simulink model "telemetrySources"  (Simulink 6.6)
settings: Solver=ode3  StartTime=0.0  StopTime=time(end)  FixedStep=0.01  RelTol=1e-3
values from neighbouring files (symbols this model uses):
  baseHeight = GPS_hil(1,3)    [telemetryToHil.m]
  GS_location = [0 36.9898376464844 -122.051963806152]    [telemetryToHil.m]
  ISA_rho0 = 1.225    [Taxi_Var.m]
  T = 0.01    [Taxi_Var.m]
undefined symbols (not defined in the file or in its folder): baroMeanTemp, baroOffset, baroScale, baroTempK, baseTemp, gaind, lapseRate, magMeanTemp, magOffset, magScale, magTempK, pitMeanTemp, pitotOffset, pitotScale, pitTempK, polesd, tempOffset, tempScale, zerosd
libraries: simulink x4, aerolibconvert2 x1
settings Model: Creator=Administrator  LastModifiedBy=Administrator

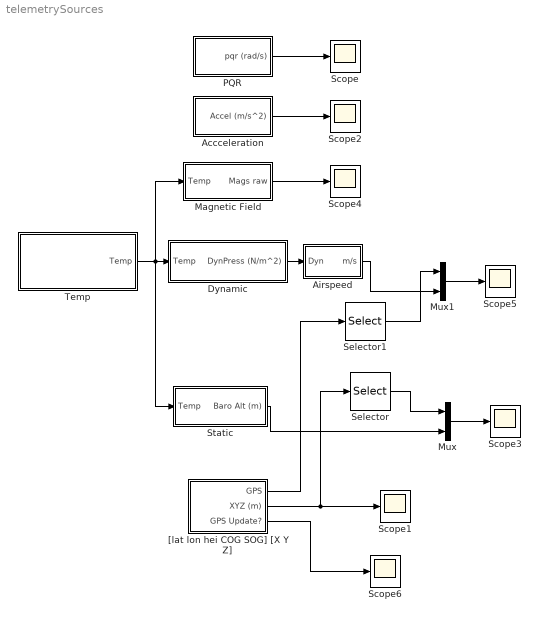
== system telemetrySources ==
  Accceleration : Subsystem
  Airspeed : Subsystem
  Dynamic : Subsystem
  Magnetic Field : Subsystem
  Mux : Mux  Inputs=2
  Mux1 : Mux  Inputs=2
  PQR : Subsystem
  Scope{,1..6} (7 alike) : Scope
      Scope1 settings: TimeRange=60  YMin=-1500  YMax=1500
      Scope2 settings: SaveName=ScopeData2
      Scope3 settings: TimeRange=1540.45  YMin=70  YMax=260  SaveName=ScopeData3
      Scope4 settings: SaveName=ScopeData4
      Scope5 settings: TimeRange=500  YMin=-40  YMax=30  SaveName=ScopeData5
      Scope6 settings: TimeRange=60  YMin=-1500  YMax=1500  SaveName=ScopeData6
  Selector : Selector  IndexOptions=Index vector (dialog)  Indices=[3]  OutputSizes=1  InputPortWidth=3
  Selector1 : Selector  IndexOptions=Index vector (dialog)  Indices=[5]  OutputSizes=1  InputPortWidth=5
  Static : Subsystem
  Temp : Subsystem
  "[lat lon hei COG SOG] [X Y Z]" : Subsystem
  wires:
  PQR/1(pqr (rad/s)) -> Scope/1
  "[lat lon hei COG SOG] [X Y Z]"/2(XYZ (m)) -> Selector/1, Scope1/1
  Accceleration/1(Accel (m/s^2)) -> Scope2/1
  Static/1(Baro Alt (m)) -> Mux/2
  Mux/1 -> Scope3/1
  Selector/1 -> Mux/1
  Magnetic Field/1(Mags raw) -> Scope4/1
  Temp/1(Temp) -> Magnetic Field/1(Temp), Dynamic/1(Temp), Static/1(Temp)
  Dynamic/1(DynPress (N/m^2)) -> Airspeed/1(Dyn)
  "[lat lon hei COG SOG] [X Y Z]"/1(GPS) -> Selector1/1
  Selector1/1 -> Mux1/1
  Mux1/1 -> Scope5/1
  Airspeed/1(m/s) -> Mux1/2
  "[lat lon hei COG SOG] [X Y Z]"/3(GPS Update?) -> Scope6/1

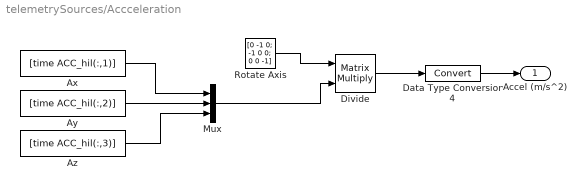
== system telemetrySources/Accceleration ==
  Ax : FromWorkspace  VariableName=[time ACC_hil(:,1)]  SampleTime=0.01  OutputAfterFinalValue=Setting to zero
  Ay : FromWorkspace  VariableName=[time ACC_hil(:,2)]  SampleTime=0.01  OutputAfterFinalValue=Setting to zero
  Az : FromWorkspace  VariableName=[time ACC_hil(:,3)]  SampleTime=0.01  OutputAfterFinalValue=Setting to zero
  Data Type Conversion4 : DataTypeConversion  OutDataTypeMode=single
  Divide : Product  Multiplication=Matrix(*)  OutScaling=2^-10
  Mux : Mux  Inputs=3
  Rotate Axis : Constant  Value=[0 -1 0; -1 0 0; 0 0 -1]
  Accel (m/s^2) : Outport
  wires:
  Az/1 -> Mux/3
  Ay/1 -> Mux/2
  Ax/1 -> Mux/1
  Data Type Conversion4/1 -> Accel (m/s^2)/1
  Rotate Axis/1 -> Divide/1
  Mux/1 -> Divide/2
  Divide/1 -> Data Type Conversion4/1

== system telemetrySources/Airspeed ==
  Dyn : Inport
  Gain : Gain  Gain=2/ISA_rho0
  Math Function : Math  Operator=sqrt  SaturateOnIntegerOverflow=on
  "[0.001  2000]" : Saturate  UpperLimit=2000  LowerLimit=0.001
  m/s : Outport
  wires:
  Gain/1 -> "[0.001  2000]"/1
  Dyn/1 -> Gain/1
  Math Function/1 -> m/s/1
  "[0.001  2000]"/1 -> Math Function/1

== system telemetrySources/Dynamic ==
  Temp : Inport
  Data Type Conversion1 : DataTypeConversion  OutDataTypeMode=single
  Dyn : FromWorkspace  VariableName=[time DYN_hil(:,1)]  SampleTime=0.01  OutputAfterFinalValue=Setting to zero
  Low Pass1 : Subsystem  mask(DiscretizedZeroPole){Zeros=[], Poles=[-30], Gain=30, AbsTol=auto, SampleTime=T, method=tustin, Wc=1}
      mask prompts: Zeros "Zeros (enter in s-main:)"; Poles "Poles (enter in s-domain:)"; Gain "Gain (enter in s-domain:)"; AbsTol "Absolute tolerance:"; SampleTime "Sample time:"; Wc "Critical Frequency (Hz):"
      mask help: Continuous mask uses c2d to transform parameters onto the Discrete Zero-Pole block inside.
      mask init:
      | st=SampleTime;
      | if length(st)>1
      |     st=SampleTime(1);
      | end
      | if(st>0)
      |     [zerosd,polesd,gaind] = sldiscutil('disczpk', {st,method,Wc,Zeros,Poles,Gain});
      | end	
      | s = get_param(gcb,'maskvalues');
      | zeross = s{1};
      | poless = s{2};
      | gainss = s{3};
      | %zerosc = eval(zeross);
      | %polesc = eval(poless);
      | %gainsc = eval(gainss);
      | sldiscutil('initzpkmask', st);
      | if(st==0)
      | set_param([gcb '/Zero Pole'], 'AbsoluteTolerance', AbsTol);
      | end
      mask StyleString: edit,edit,edit,edit,edit,popup(zoh|foh|tustin|prewarp|matched),edit
      mask CallbackString: |||||hidecrit|
      mask Display:
      | droots(zeross,poless,gainss)
      | text( 0.5, 1.0, method, 'verticalAlignment','top')
  Pitot Unit Conversion : Subsystem  mask{bias=pitotOffset, gains=pitotScale}
      mask prompts: bias "Initial Bias"; gains "Initial Gains"
      mask help: Convert Analog readings to units
  Pitot Temp Compensation : Subsystem  mask{alpha=pitTempK, tempMean=pitMeanTemp}
      mask prompts: alpha "Tempearature Coeficient (K_t)"; tempMean "Calibration Temperature Mean (T_avg)"
      mask help:
      | This block implements a temperature compensation. It implmements the following equation:
      |
      | M_tc = M_raw - K_t(T - T_avg)
  DynPress (N/m^2) : Outport
  wires:
  Dyn/1 -> Low Pass1/1(In1)
  Low Pass1/1(Out1) -> Data Type Conversion1/1
  Data Type Conversion1/1 -> Pitot Unit Conversion/1(Raw)
  Pitot Temp Compensation/1(Comp) -> DynPress (N/m^2)/1
  Temp/1 -> Pitot Temp Compensation/2(Temp Raw)
  Pitot Unit Conversion/1(Comp) -> Pitot Temp Compensation/1(Raw)

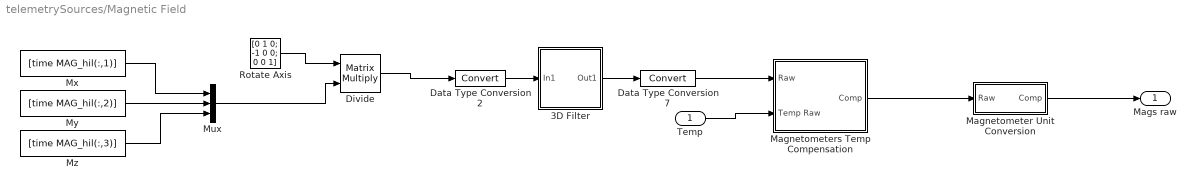
== system telemetrySources/Magnetic Field ==
  Temp : Inport
  3D Filter : Subsystem  AncestorBlock=SLUGS_Library/Singnal Routing & Conditioning/3D Filter  RTWFcnName=TustinFilter3D  mask{zval=[], pval=-150, kval=150, TSample=0.01}
      mask prompts: zval "Zeros"; pval "Poles"; kval "Gains"; TSample "Sample Time"
      settings: RTWFcnNameOpts=User specified  RTWFileNameOpts=Use function name
      mask Display:
      | droots(zval,pval,kval)
      | port_label('input',1,'3D')
  Data Type Conversion2 : DataTypeConversion  OutDataTypeMode=double
  Data Type Conversion7 : DataTypeConversion  OutDataTypeMode=single
  Divide : Product  Multiplication=Matrix(*)  OutScaling=2^-10
  Magnetometer Unit Conversion : Subsystem  mask{bias=magOffset, gains=magScale}
      mask prompts: bias "Initial Bias"; gains "Initial Gains"
      mask help: Convert Analog readings to units
  Magnetometers Temp Compensation : Subsystem  mask{alpha=magTempK, tempMean=magMeanTemp}
      mask prompts: alpha "Tempearature Coeficient (K_t)"; tempMean "Calibration Temperature Mean (T_avg)"
      mask help:
      | This block implements a temperature compensation. It implmements the following equation:
      |
      | M_tc = M_raw - K_t(T - T_avg)
  Mux : Mux  Inputs=3
  Mx : FromWorkspace  VariableName=[time MAG_hil(:,1)]  SampleTime=0.01  OutputAfterFinalValue=Setting to zero
  My : FromWorkspace  VariableName=[time MAG_hil(:,2)]  SampleTime=0.01  OutputAfterFinalValue=Setting to zero
  Mz : FromWorkspace  VariableName=[time MAG_hil(:,3)]  SampleTime=0.01  OutputAfterFinalValue=Setting to zero
  Rotate Axis : Constant  Value=[0 1 0; -1 0 0; 0 0 1]
  Mags raw : Outport
  wires:
  Mx/1 -> Mux/1
  My/1 -> Mux/2
  Mz/1 -> Mux/3
  Rotate Axis/1 -> Divide/1
  Mux/1 -> Divide/2
  Data Type Conversion2/1 -> 3D Filter/1(In1)
  3D Filter/1(Out1) -> Data Type Conversion7/1
  Data Type Conversion7/1 -> Magnetometers Temp Compensation/1(Raw)
  Magnetometers Temp Compensation/1(Comp) -> Magnetometer Unit Conversion/1(Raw)
  Divide/1 -> Data Type Conversion2/1
  Temp/1 -> Magnetometers Temp Compensation/2(Temp Raw)
  Magnetometer Unit Conversion/1(Comp) -> Mags raw/1

== system telemetrySources/PQR ==
  Data Type Conversion1 : DataTypeConversion  OutDataTypeMode=single
  Divide : Product  Multiplication=Matrix(*)  OutScaling=2^-10
  Mux : Mux  Inputs=3
  Rotate Axis : Constant  Value=[0 -1 0; -1 0 0; 0 0 -1]
  p : FromWorkspace  VariableName=[time PQR_hil(:,1)]  SampleTime=0.01  OutputAfterFinalValue=Setting to zero
  q : FromWorkspace  VariableName=[time PQR_hil(:,2)]  SampleTime=0.01  OutputAfterFinalValue=Setting to zero
  r : FromWorkspace  VariableName=[time PQR_hil(:,3)]  SampleTime=0.01  OutputAfterFinalValue=Setting to zero
  pqr (rad/s) : Outport
  wires:
  p/1 -> Mux/1
  q/1 -> Mux/2
  r/1 -> Mux/3
  Data Type Conversion1/1 -> pqr (rad/s)/1
  Rotate Axis/1 -> Divide/1
  Mux/1 -> Divide/2
  Divide/1 -> Data Type Conversion1/1

== system telemetrySources/Static ==
  Temp : Inport
  Baro Altimeter : Subsystem
  Baro Temp Compensation : Subsystem  mask{alpha=baroTempK, tempMean=baroMeanTemp}
      mask prompts: alpha "Tempearature Coeficient (K_t)"; tempMean "Calibration Temperature Mean (T_avg)"
      mask help:
      | This block implements a temperature compensation. It implmements the following equation:
      |
      | M_tc = M_raw - K_t(T - T_avg)
  Barometer Unit Conversion : Subsystem  mask{bias=baroOffset, gains=baroScale}
      mask prompts: bias "Initial Bias"; gains "Initial Gains"
      mask help: Convert Analog readings to units
  Data Type Conversion1 : DataTypeConversion  OutDataTypeMode=single
  Dyn : FromWorkspace  VariableName=[time STA_hil(:,1)]  SampleTime=0.01  OutputAfterFinalValue=Setting to zero
  Low Pass1 : Subsystem  mask(DiscretizedZeroPole){Zeros=[], Poles=[-1], Gain=1, AbsTol=auto, SampleTime=T, method=tustin, Wc=1}
      mask prompts: Zeros "Zeros (enter in s-main:)"; Poles "Poles (enter in s-domain:)"; Gain "Gain (enter in s-domain:)"; AbsTol "Absolute tolerance:"; SampleTime "Sample time:"; Wc "Critical Frequency (Hz):"
      mask help: Continuous mask uses c2d to transform parameters onto the Discrete Zero-Pole block inside.
      mask init: same as telemetrySources/Dynamic/Low Pass1
      mask StyleString: edit,edit,edit,edit,edit,popup(zoh|foh|tustin|prewarp|matched),edit
      mask CallbackString: |||||hidecrit|
      mask Display:
      | droots(zeross,poless,gainss)
      | text( 0.5, 1.0, method, 'verticalAlignment','top')
  Baro Alt (m) : Outport
  wires:
  Low Pass1/1(Out1) -> Data Type Conversion1/1
  Dyn/1 -> Low Pass1/1(In1)
  Baro Altimeter/1(Altitude) -> Baro Alt (m)/1
  Barometer Unit Conversion/1(Comp) -> Baro Temp Compensation/1(Raw)
  Baro Temp Compensation/1(Comp) -> Baro Altimeter/1(Static Raw)
  Data Type Conversion1/1 -> Barometer Unit Conversion/1(Raw)
  Temp/1 -> Baro Temp Compensation/2(Temp Raw)

== system telemetrySources/Temp ==
  Data Type Conversion5 : DataTypeConversion  OutDataTypeMode=single
  Dyn : FromWorkspace  VariableName=[time TEM_hil(:,1)]  SampleTime=0.01  OutputAfterFinalValue=Setting to zero
  Low Pass8 : Subsystem  mask(DiscretizedZeroPole){Zeros=[], Poles=[-5], Gain=5, AbsTol=auto, SampleTime=T, method=tustin, Wc=1}
      mask prompts: Zeros "Zeros (enter in s-main:)"; Poles "Poles (enter in s-domain:)"; Gain "Gain (enter in s-domain:)"; AbsTol "Absolute tolerance:"; SampleTime "Sample time:"; Wc "Critical Frequency (Hz):"
      mask help: Continuous mask uses c2d to transform parameters onto the Discrete Zero-Pole block inside.
      mask init: same as telemetrySources/Dynamic/Low Pass1
      mask StyleString: edit,edit,edit,edit,edit,popup(zoh|foh|tustin|prewarp|matched),edit
      mask CallbackString: |||||hidecrit|
      mask Display:
      | droots(zeross,poless,gainss)
      | text( 0.5, 1.0, method, 'verticalAlignment','top')
  Thermistor Unit Conversion : Subsystem  mask{bias=tempOffset, gains=tempScale}
      mask prompts: bias "Initial Bias"; gains "Initial Gains"
      mask help: Convert Analog readings to units
  Temp : Outport
  wires:
  Dyn/1 -> Low Pass8/1(In1)
  Low Pass8/1(Out1) -> Data Type Conversion5/1
  Thermistor Unit Conversion/1(Comp) -> Temp/1
  Data Type Conversion5/1 -> Thermistor Unit Conversion/1(Raw)

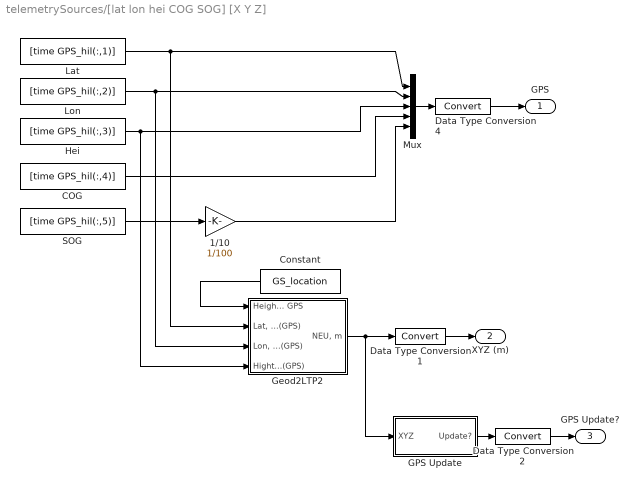
== system telemetrySources/[lat lon hei COG SOG] [X Y Z] ==
  1/10 : Gain  Gain=1/100
  COG : FromWorkspace  VariableName=[time GPS_hil(:,4)]  SampleTime=0.01  OutputAfterFinalValue=Setting to zero
  Constant : Constant  Orientation=left  Value=GS_location
  Data Type Conversion1 : DataTypeConversion  OutDataTypeMode=single
  Data Type Conversion2 : DataTypeConversion  OutDataTypeMode=uint8
  Data Type Conversion4 : DataTypeConversion  OutDataTypeMode=single
  GPS Update : Subsystem  mask{T=0.01}
      mask prompts: T "Sample Time"
  Geod2LTP2 : Subsystem
      mask Description:
      | This block provides transformation of the Geodetic coordinates
      | to the LTP coorinate system. The block uses two consecutive transformations
      | (Geodetic -> ECEF ->LTP).
      | Geodetic coordinates of the LTP origin should also be predetermined.
      mask Help: Oops!
      mask Display: plot(0,0,100,100,[45,40,35,40,40],[85,95,85,95,40],[85,95,85,95,40],[35,40,45,40,40],[60,40,10,20,10,14],[70,40,10,13,10,20],[56,45],[70,70],[60,60],[50,60],[60,60],[30,40],[50,60],[20,20],[30,40],[20,20],[45,55],[35,25],[75,65],[35,25])
  Hei : FromWorkspace  VariableName=[time GPS_hil(:,3)]  SampleTime=0.01  OutputAfterFinalValue=Setting to zero
  Lat : FromWorkspace  VariableName=[time GPS_hil(:,1)]  SampleTime=0.01  OutputAfterFinalValue=Setting to zero
  Lon : FromWorkspace  VariableName=[time GPS_hil(:,2)]  SampleTime=0.01  OutputAfterFinalValue=Setting to zero
  Mux : Mux  Inputs=5
  SOG : FromWorkspace  VariableName=[time GPS_hil(:,5)]  SampleTime=0.01  OutputAfterFinalValue=Setting to zero
  GPS : Outport
  XYZ (m) : Outport  Port=2
  GPS Update? : Outport  Port=3
  wires:
  Lat/1 -> Mux/1, Geod2LTP2/2("Lat, deg(GPS)")
  Lon/1 -> Mux/2, Geod2LTP2/3("Lon, deg(GPS)")
  Hei/1 -> Mux/3, Geod2LTP2/4(Hight,m(GPS))
  Mux/1 -> Data Type Conversion4/1
  COG/1 -> Mux/4
  SOG/1 -> 1/10/1
  Constant/1 -> Geod2LTP2/1("Height, Lat, Lon Initials from GPS")
  Geod2LTP2/1("NEU, m") -> GPS Update/1(XYZ), Data Type Conversion1/1
  GPS Update/1(Update?) -> Data Type Conversion2/1
  1/10/1 -> Mux/5
  Data Type Conversion4/1 -> GPS/1
  Data Type Conversion1/1 -> XYZ (m)/1
  Data Type Conversion2/1 -> GPS Update?/1

== system telemetrySources/Dynamic/Low Pass1 ==
  In1 : Inport
  Discrete Zero-Pole : DiscreteZeroPole  Zeros=zerosd  Poles=polesd  Gain=gaind  SampleTime=SampleTime
  Out1 : Outport
  wires:
  In1/1 -> Discrete Zero-Pole/1
  Discrete Zero-Pole/1 -> Out1/1

== system telemetrySources/Dynamic/Pitot Unit Conversion ==
  Raw : Inport
  Bias : Constant  Value=bias  OutDataTypeMode=single
  Divide : Product  OutDataTypeMode=single  OutScaling=2^-10
  Gains : Constant  Value=gains  OutDataTypeMode=single
  Sum : Sum  Inputs=|++  OutDataTypeMode=single
  Comp : Outport
  wires:
  Bias/1 -> Sum/2
  Raw/1 -> Divide/2
  Gains/1 -> Divide/1
  Divide/1 -> Sum/1
  Sum/1 -> Comp/1

== system telemetrySources/Dynamic/Pitot Temp Compensation ==
  Raw : Inport
  Temp Raw : Inport  Port=2
  Divide1 : Product  OutDataTypeMode=single  OutScaling=2^-10
  Mean Temperature for Calibration : Constant  Value=tempMean  OutDataTypeMode=single
  Sum1 : Sum  Inputs=|+-  OutDataTypeMode=single
  Sum2 : Sum  Inputs=|+-  OutDataTypeMode=single
  gains : Constant  Value=alpha  OutDataTypeMode=single
  Comp : Outport
  wires:
  Mean Temperature for Calibration/1 -> Sum1/2
  Raw/1 -> Sum2/1
  Temp Raw/1 -> Sum1/1
  Sum1/1 -> Divide1/2
  gains/1 -> Divide1/1
  Divide1/1 -> Sum2/2
  Sum2/1 -> Comp/1

== system telemetrySources/Magnetic Field/3D Filter ==
  In1 : Inport
  Demux : Demux  Outputs=3
  Filter1 : Subsystem  mask(DiscretizedZeroPole){Zeros=zval, Poles=pval, Gain=kval, AbsTol=auto, SampleTime=TSample, method=tustin, Wc=1}
      mask prompts: Zeros "Zeros (enter in s-main:)"; Poles "Poles (enter in s-domain:)"; Gain "Gain (enter in s-domain:)"; AbsTol "Absolute tolerance:"; SampleTime "Sample time:"; Wc "Critical Frequency (Hz):"
      mask help: Continuous mask uses c2d to transform parameters onto the Discrete Zero-Pole block inside.
      mask init: same as telemetrySources/Dynamic/Low Pass1
      mask StyleString: edit,edit,edit,edit,edit,popup(zoh|foh|tustin|prewarp|matched),edit
      mask CallbackString: |||||hidecrit|
      mask Display:
      | droots(zeross,poless,gainss)
      | text( 0.5, 1.0, method, 'verticalAlignment','top')
  Filter2 : Subsystem  mask(DiscretizedZeroPole){Zeros=zval, Poles=pval, Gain=kval, AbsTol=auto, SampleTime=TSample, method=tustin, Wc=1}
      mask prompts: Zeros "Zeros (enter in s-main:)"; Poles "Poles (enter in s-domain:)"; Gain "Gain (enter in s-domain:)"; AbsTol "Absolute tolerance:"; SampleTime "Sample time:"; Wc "Critical Frequency (Hz):"
      mask help: Continuous mask uses c2d to transform parameters onto the Discrete Zero-Pole block inside.
      mask init: same as telemetrySources/Dynamic/Low Pass1
      mask StyleString: edit,edit,edit,edit,edit,popup(zoh|foh|tustin|prewarp|matched),edit
      mask CallbackString: |||||hidecrit|
      mask Display:
      | droots(zeross,poless,gainss)
      | text( 0.5, 1.0, method, 'verticalAlignment','top')
  Filter3 : Subsystem  mask(DiscretizedZeroPole){Zeros=zval, Poles=pval, Gain=kval, AbsTol=auto, SampleTime=TSample, method=tustin, Wc=1}
      mask prompts: Zeros "Zeros (enter in s-main:)"; Poles "Poles (enter in s-domain:)"; Gain "Gain (enter in s-domain:)"; AbsTol "Absolute tolerance:"; SampleTime "Sample time:"; Wc "Critical Frequency (Hz):"
      mask help: Continuous mask uses c2d to transform parameters onto the Discrete Zero-Pole block inside.
      mask init: same as telemetrySources/Dynamic/Low Pass1
      mask StyleString: edit,edit,edit,edit,edit,popup(zoh|foh|tustin|prewarp|matched),edit
      mask CallbackString: |||||hidecrit|
      mask Display:
      | droots(zeross,poless,gainss)
      | text( 0.5, 1.0, method, 'verticalAlignment','top')
  myMux Fun1 : Stateflow chart
  Out1 : Outport
  wires:
  myMux Fun1/1(y) -> Out1/1
  In1/1 -> Demux/1
  Filter3/1(Out1) -> myMux Fun1/3(u3)
  Filter2/1(Out1) -> myMux Fun1/2(u2)
  Filter1/1(Out1) -> myMux Fun1/1(u1)
  Demux/3 -> Filter3/1(In1)
  Demux/2 -> Filter2/1(In1)
  Demux/1 -> Filter1/1(In1)

== system telemetrySources/Magnetic Field/Magnetometer Unit Conversion ==
  Raw : Inport
  Bias : Constant  Value=bias  OutDataTypeMode=single
  Divide : Product  OutDataTypeMode=single  OutScaling=2^-10
  Gains : Constant  Value=gains  OutDataTypeMode=single
  Sum : Sum  Inputs=|++  OutDataTypeMode=single
  Comp : Outport
  wires:
  Bias/1 -> Sum/2
  Raw/1 -> Divide/2
  Gains/1 -> Divide/1
  Divide/1 -> Sum/1
  Sum/1 -> Comp/1

== system telemetrySources/Magnetic Field/Magnetometers Temp Compensation ==
  Raw : Inport
  Temp Raw : Inport  Port=2
  Divide1 : Product  OutDataTypeMode=single  OutScaling=2^-10
  Mean Temperature for Calibration : Constant  Value=tempMean  OutDataTypeMode=single
  Sum1 : Sum  Inputs=|+-  OutDataTypeMode=single
  Sum2 : Sum  Inputs=|+-  OutDataTypeMode=single
  gains : Constant  Value=alpha  OutDataTypeMode=single
  Comp : Outport
  wires:
  Sum2/1 -> Comp/1
  Divide1/1 -> Sum2/2
  gains/1 -> Divide1/1
  Sum1/1 -> Divide1/2
  Temp Raw/1 -> Sum1/1
  Raw/1 -> Sum2/1
  Mean Temperature for Calibration/1 -> Sum1/2

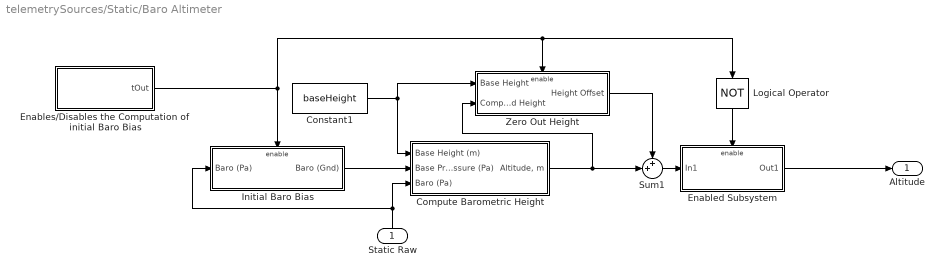
== system telemetrySources/Static/Baro Altimeter ==
  Static Raw : Inport  Orientation=up
  Compute Barometric Height : Subsystem  mask{baseTemp=baseTemp, LapseRate=lapseRate}
      mask prompts: baseTemp "Base Station Temperature (K)"; LapseRate "Lapse Rate (C/ft)"
      mask help:
      | Produces Altitude in meters from Barometric Pressure in Pascals. Altitude is valid from MSL to 6000 ft.
      |
      | The method implemented here was developed by Ren Curry
  Constant1 : Constant  Value=baseHeight  OutDataTypeMode=single
  Enabled Subsystem : Subsystem  TreatAsAtomicUnit=on
  Enables/Disables the Computation of  initial Baro Bias : Stateflow chart
  Initial Baro Bias : Subsystem  TreatAsAtomicUnit=on
  Logical Operator : Logic  Orientation=down  Operator=NOT  AllPortsSameDT=off  OutDataTypeMode=Boolean
  Sum1 : Sum  Inputs=++|  OutDataTypeMode=single
  Zero Out Height : Subsystem  TreatAsAtomicUnit=on
  Altitude : Outport
  wires:
  Compute Barometric Height/1("Altitude, m") -> Zero Out Height/2(Computed Height), Sum1/2
  Static Raw/1 -> Initial Baro Bias/1(Baro (Pa)), Compute Barometric Height/3(Baro (Pa))
  Enables/Disables the Computation of  initial Baro Bias/1(tOut) -> Initial Baro Bias/Enable, Zero Out Height/Enable, Logical Operator/1
  Constant1/1 -> Compute Barometric Height/1(Base Height (m)), Zero Out Height/1(Base Height)
  Initial Baro Bias/1(Baro (Gnd)) -> Compute Barometric Height/2(Base Pressure (Pa))
  Zero Out Height/1(Height Offset) -> Sum1/1
  Sum1/1 -> Enabled Subsystem/1(In1)
  Enabled Subsystem/1(Out1) -> Altitude/1
  Logical Operator/1 -> Enabled Subsystem/Enable

== system telemetrySources/Static/Baro Temp Compensation ==
  Raw : Inport
  Temp Raw : Inport  Port=2
  Divide1 : Product  OutDataTypeMode=single  OutScaling=2^-10
  Mean Temperature for Calibration : Constant  Value=tempMean  OutDataTypeMode=single
  Sum1 : Sum  Inputs=|+-  OutDataTypeMode=single
  Sum2 : Sum  Inputs=|+-  OutDataTypeMode=single
  gains : Constant  Value=alpha  OutDataTypeMode=single
  Comp : Outport
  wires:
  Mean Temperature for Calibration/1 -> Sum1/2
  Raw/1 -> Sum2/1
  Temp Raw/1 -> Sum1/1
  Sum1/1 -> Divide1/2
  gains/1 -> Divide1/1
  Divide1/1 -> Sum2/2
  Sum2/1 -> Comp/1

== system telemetrySources/Static/Barometer Unit Conversion ==
  Raw : Inport
  Bias : Constant  Value=bias  OutDataTypeMode=single
  Divide : Product  OutDataTypeMode=single  OutScaling=2^-10
  Gains : Constant  Value=gains  OutDataTypeMode=single
  Sum : Sum  Inputs=|++  OutDataTypeMode=single
  Comp : Outport
  wires:
  Bias/1 -> Sum/2
  Raw/1 -> Divide/2
  Gains/1 -> Divide/1
  Divide/1 -> Sum/1
  Sum/1 -> Comp/1

== system telemetrySources/Static/Low Pass1 ==
  In1 : Inport
  Discrete Zero-Pole : DiscreteZeroPole  Zeros=zerosd  Poles=polesd  Gain=gaind  SampleTime=SampleTime
  Out1 : Outport
  wires:
  Discrete Zero-Pole/1 -> Out1/1
  In1/1 -> Discrete Zero-Pole/1

== system telemetrySources/Temp/Low Pass8 ==
  In1 : Inport
  Discrete Zero-Pole : DiscreteZeroPole  Zeros=zerosd  Poles=polesd  Gain=gaind  SampleTime=SampleTime
  Out1 : Outport
  wires:
  In1/1 -> Discrete Zero-Pole/1
  Discrete Zero-Pole/1 -> Out1/1

== system telemetrySources/Temp/Thermistor Unit Conversion ==
  Raw : Inport
  Bias : Constant  Value=bias  OutDataTypeMode=single
  Divide : Product  OutDataTypeMode=single  OutScaling=2^-10
  Gains : Constant  Value=gains  OutDataTypeMode=single
  Sum : Sum  Inputs=|++  OutDataTypeMode=single
  Comp : Outport
  wires:
  Sum/1 -> Comp/1
  Divide/1 -> Sum/1
  Gains/1 -> Divide/1
  Raw/1 -> Divide/2
  Bias/1 -> Sum/2

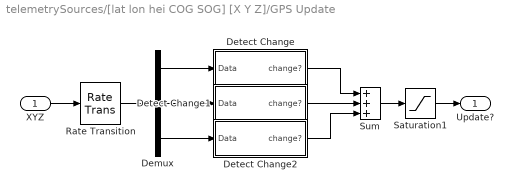
== system telemetrySources/[lat lon hei COG SOG] [X Y Z]/GPS Update ==
  XYZ : Inport
  Demux : Demux  Outputs=3
  Detect Change : Subsystem
  Detect Change1 : Subsystem
  Detect Change2 : Subsystem
  Rate Transition : RateTransition  OutPortSampleTime=T
  Saturation1 : Saturate  UpperLimit=1  LowerLimit=0  SampleTime=T
  Sum : Sum  Inputs=3
  Update? : Outport
  wires:
  Demux/1 -> Detect Change/1(Data)
  Demux/2 -> Detect Change1/1(Data)
  Demux/3 -> Detect Change2/1(Data)
  Detect Change/1(change?) -> Sum/1
  Detect Change1/1(change?) -> Sum/2
  Detect Change2/1(change?) -> Sum/3
  Sum/1 -> Saturation1/1
  XYZ/1 -> Rate Transition/1
  Saturation1/1 -> Update?/1
  Rate Transition/1 -> Demux/1

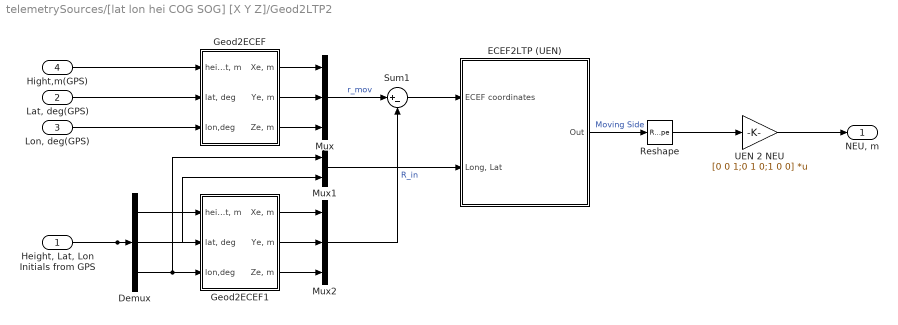
== system telemetrySources/[lat lon hei COG SOG] [X Y Z]/Geod2LTP2 ==
  "Height, Lat, Lon Initials from GPS" : Inport
  "Lat, deg(GPS)" : Inport  Port=2
  "Lon, deg(GPS)" : Inport  Port=3
  Hight,m(GPS) : Inport  Port=4
  Demux : Demux  Outputs=3
  ECEF2LTP (UEN) : Subsystem
      mask Display: plot(0,0,100,100,[45,40,35,40,40],[85,95,85,95,40],[85,95,85,95,40],[35,40,45,40,40],[60,40,10,20,10,14],[70,40,10,13,10,20],[56,45],[70,70],[60,60],[50,60],[60,60],[30,40],[50,60],[20,20],[30,40],[20,20],[45,55],[35,25],[75,65],[35,25])
  Geod2ECEF : Subsystem  mask{Re=6378137, Rp=6356752.3142}
      mask prompts: Re "Enter equatorial radius, m"; Rp "Enter polar radius,m"
  Geod2ECEF1 : Subsystem  mask{Re=6378137, Rp=6356752.3142}
      mask prompts: Re "Enter equatorial radius, m"; Rp "Enter polar radius,m"
  Mux : Mux  Inputs=3
  Mux1 : Mux  Inputs=2
  Mux2 : Mux  Inputs=3
  Reshape : Reshape  OutputDimensionality=Column vector (2-D)
  Sum1 : Sum  Inputs=|+-  SaturateOnIntegerOverflow=on
  UEN 2 NEU : Gain  Gain=[0 0 1;0 1 0;1 0 0]  Multiplication=Matrix(K*u)  SaturateOnIntegerOverflow=on
  "NEU, m" : Outport
  wires:
  UEN 2 NEU/1 -> "NEU, m"/1
  Geod2ECEF/3("Ze, m ") -> Mux/3
  Geod2ECEF/1("Xe, m ") -> Mux/1
  Geod2ECEF/2("Ye, m ") -> Mux/2
  "Lat, deg(GPS)"/1 -> Geod2ECEF/2("lat, deg")
  "Lon, deg(GPS)"/1 -> Geod2ECEF/3(lon,deg)
  Mux1/1 -> ECEF2LTP (UEN)/2("Long, Lat")
  Geod2ECEF1/3("Ze, m ") -> Mux2/3
  Geod2ECEF1/1("Xe, m ") -> Mux2/1
  Geod2ECEF1/2("Ye, m ") -> Mux2/2
  Mux2/1 -> Sum1/2  "R_in"
  Demux/1 -> Geod2ECEF1/1("height, m")
  Demux/2 -> Mux1/2, Geod2ECEF1/2("lat, deg")
  Demux/3 -> Mux1/1, Geod2ECEF1/3(lon,deg)
  ECEF2LTP (UEN)/1(Out) -> Reshape/1  "Moving Side"
  Hight,m(GPS)/1 -> Geod2ECEF/1("height, m")
  "Height, Lat, Lon Initials from GPS"/1 -> Demux/1
  Mux/1 -> Sum1/1  "r_mov"
  Sum1/1 -> ECEF2LTP (UEN)/1(ECEF coordinates)
  Reshape/1 -> UEN 2 NEU/1

== system telemetrySources/Magnetic Field/3D Filter/Filter1 ==
  In1 : Inport
  Discrete Zero-Pole : DiscreteZeroPole  Zeros=zerosd  Poles=polesd  Gain=gaind  SampleTime=SampleTime
  Out1 : Outport
  wires:
  Discrete Zero-Pole/1 -> Out1/1
  In1/1 -> Discrete Zero-Pole/1

== system telemetrySources/Magnetic Field/3D Filter/Filter2 ==
  In1 : Inport
  Discrete Zero-Pole : DiscreteZeroPole  Zeros=zerosd  Poles=polesd  Gain=gaind  SampleTime=SampleTime
  Out1 : Outport
  wires:
  In1/1 -> Discrete Zero-Pole/1
  Discrete Zero-Pole/1 -> Out1/1

== system telemetrySources/Magnetic Field/3D Filter/Filter3 ==
  In1 : Inport
  Discrete Zero-Pole : DiscreteZeroPole  Zeros=zerosd  Poles=polesd  Gain=gaind  SampleTime=SampleTime
  Out1 : Outport
  wires:
  Discrete Zero-Pole/1 -> Out1/1
  In1/1 -> Discrete Zero-Pole/1

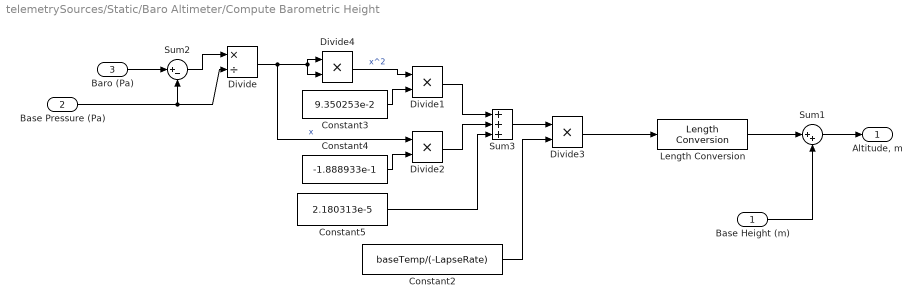
== system telemetrySources/Static/Baro Altimeter/Compute Barometric Height ==
  Base Height (m) : Inport
  Base Pressure (Pa) : Inport  Port=2
  Baro (Pa) : Inport  Port=3
  Constant2 : Constant  Value=baseTemp/(-LapseRate)  OutDataTypeMode=single
  Constant3 : Constant  Value=9.350253e-2  OutDataTypeMode=single
  Constant4 : Constant  Value=-1.888933e-1  OutDataTypeMode=single
  Constant5 : Constant  Value=2.180313e-5  OutDataTypeMode=single
  Divide : Product  Inputs=*/  OutDataTypeMode=single  OutScaling=2^-10
  Divide{1..4} (4 alike) : Product  OutDataTypeMode=single  OutScaling=2^-10
  Length Conversion : aerolibconvert2/Length Conversion  SystemSampleTime=-1  IU=ft  OU=m
  Sum1 : Sum  Inputs=|++  OutDataTypeMode=single
  Sum2 : Sum  Inputs=|+-  OutDataTypeMode=single
  Sum3 : Sum  Inputs=3  OutDataTypeMode=single
  "Altitude, m" : Outport
  wires:
  Length Conversion/1 -> Sum1/1
  Sum2/1 -> Divide/1
  Sum1/1 -> "Altitude, m"/1
  Divide3/1 -> Length Conversion/1
  Constant2/1 -> Divide3/2
  Sum3/1 -> Divide3/1
  Constant5/1 -> Sum3/3
  Divide2/1 -> Sum3/2
  Divide1/1 -> Sum3/1
  Constant4/1 -> Divide2/2
  Constant3/1 -> Divide1/2
  Divide4/1 -> Divide1/1  "x^2"
  Divide/1 -> Divide2/1, Divide4/1, Divide4/2  "x"
  Base Pressure (Pa)/1 -> Divide/2, Sum2/2
  Base Height (m)/1 -> Sum1/2
  Baro (Pa)/1 -> Sum2/1

== system telemetrySources/Static/Baro Altimeter/Enabled Subsystem ==
  In1 : Inport
  Enable : EnablePort
  Out1 : Outport  InitialOutput=baseHeight
  wires:
  In1/1 -> Out1/1

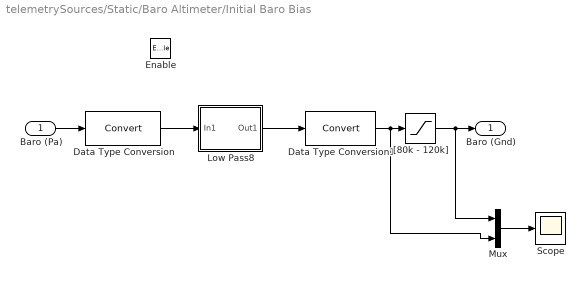
== system telemetrySources/Static/Baro Altimeter/Initial Baro Bias ==
  Baro (Pa) : Inport
  Enable : EnablePort
  Data Type Conversion : DataTypeConversion  OutDataTypeMode=double
  Data Type Conversion1 : DataTypeConversion  OutDataTypeMode=single
  Low Pass8 : Subsystem  mask(DiscretizedZeroPole){Zeros=[], Poles=[-3], Gain=3, AbsTol=auto, SampleTime=.01, method=tustin, Wc=1}
      mask prompts: Zeros "Zeros (enter in s-main:)"; Poles "Poles (enter in s-domain:)"; Gain "Gain (enter in s-domain:)"; AbsTol "Absolute tolerance:"; SampleTime "Sample time:"; Wc "Critical Frequency (Hz):"
      mask help: Continuous mask uses c2d to transform parameters onto the Discrete Zero-Pole block inside.
      mask init: same as telemetrySources/Dynamic/Low Pass1
      mask StyleString: edit,edit,edit,edit,edit,popup(zoh|foh|tustin|prewarp|matched),edit
      mask CallbackString: |||||hidecrit|
      mask Display:
      | droots(zeross,poless,gainss)
      | text( 0.5, 1.0, method, 'verticalAlignment','top')
  Mux : Mux  Inputs=2
  Scope : Scope
      settings: SaveName=ScopeData8
  "[80k - 120k]" : Saturate  UpperLimit=120000  LowerLimit=80000
  Baro (Gnd) : Outport
  wires:
  Baro (Pa)/1 -> Data Type Conversion/1
  Low Pass8/1(Out1) -> Data Type Conversion1/1
  Data Type Conversion/1 -> Low Pass8/1(In1)
  Data Type Conversion1/1 -> Mux/2, "[80k - 120k]"/1
  Mux/1 -> Scope/1
  "[80k - 120k]"/1 -> Baro (Gnd)/1, Mux/1

== system telemetrySources/Static/Baro Altimeter/Zero Out Height ==
  Base Height : Inport
  Computed Height : Inport  Port=2
  Enable : EnablePort
  Integer Delay : simulink/Discrete/Integer Delay  vinit=0  samptime=.01  NumDelays=1
  Sum : Sum  Inputs=|+-  OutDataTypeMode=single
  Height Offset : Outport
  wires:
  Computed Height/1 -> Integer Delay/1
  Sum/1 -> Height Offset/1
  Integer Delay/1 -> Sum/2
  Base Height/1 -> Sum/1

== system telemetrySources/[lat lon hei COG SOG] [X Y Z]/GPS Update/Detect Change ==
  Data : Inport
  Abs1 : Abs  SampleTime=T
  Difference1 : simulink/Discrete/Difference  SystemSampleTime=-1  ICPrevInput=0.0  OutDataType=sfix(16)  OutScaling=2^-10  DoSatur=off
  Saturation1 : Saturate  UpperLimit=1  LowerLimit=0  SampleTime=T
  change? : Outport
  wires:
  Difference1/1 -> Abs1/1
  Abs1/1 -> Saturation1/1
  Data/1 -> Difference1/1
  Saturation1/1 -> change?/1

== system telemetrySources/[lat lon hei COG SOG] [X Y Z]/GPS Update/Detect Change1 ==
  Data : Inport
  Abs1 : Abs  SampleTime=T
  Difference1 : simulink/Discrete/Difference  SystemSampleTime=-1  ICPrevInput=0.0  OutDataType=sfix(16)  OutScaling=2^-10  DoSatur=off
  Saturation1 : Saturate  UpperLimit=1  LowerLimit=0  SampleTime=T
  change? : Outport
  wires:
  Saturation1/1 -> change?/1
  Data/1 -> Difference1/1
  Abs1/1 -> Saturation1/1
  Difference1/1 -> Abs1/1

== system telemetrySources/[lat lon hei COG SOG] [X Y Z]/GPS Update/Detect Change2 ==
  Data : Inport
  Abs1 : Abs  SampleTime=T
  Difference1 : simulink/Discrete/Difference  SystemSampleTime=-1  ICPrevInput=0.0  OutDataType=sfix(16)  OutScaling=2^-10  DoSatur=off
  Saturation1 : Saturate  UpperLimit=1  LowerLimit=0  SampleTime=T
  change? : Outport
  wires:
  Difference1/1 -> Abs1/1
  Abs1/1 -> Saturation1/1
  Data/1 -> Difference1/1
  Saturation1/1 -> change?/1

== system telemetrySources/[lat lon hei COG SOG] [X Y Z]/Geod2LTP2/ECEF2LTP (UEN) ==
  ECEF coordinates : Inport
  "Long, Lat" : Inport  Port=2
  Deg2R : Gain  Gain=pi/180  SaturateOnIntegerOverflow=on
  Demux3 : Demux  Outputs=2
  From Body to Universal1 : Subsystem
  Product1 : Product  Multiplication=Matrix(*)  SaturateOnIntegerOverflow=on  InputSameDT=on
  Out : Outport
  wires:
  "Long, Lat"/1 -> Deg2R/1
  Product1/1 -> Out/1
  Demux3/2 -> From Body to Universal1/2(lat)
  Demux3/1 -> From Body to Universal1/1(long)
  Deg2R/1 -> Demux3/1
  ECEF coordinates/1 -> Product1/2
  From Body to Universal1/1(DCM) -> Product1/1

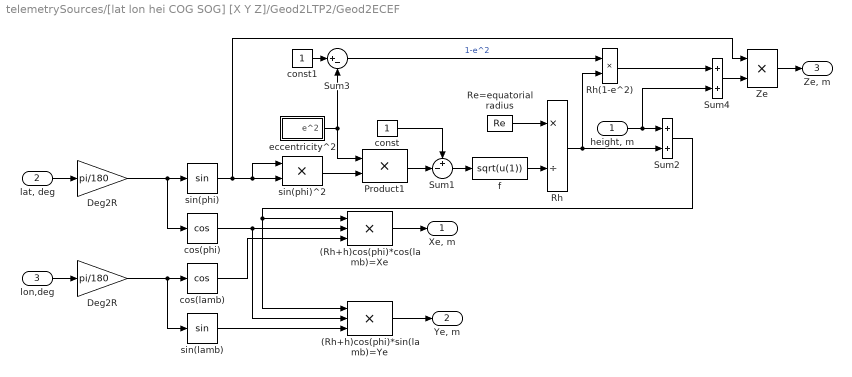
== system telemetrySources/[lat lon hei COG SOG] [X Y Z]/Geod2LTP2/Geod2ECEF ==
  "height, m" : Inport
  "lat, deg" : Inport  Port=2
  lon,deg : Inport  Port=3
  (Rh+h)cos(phi)*cos(lamb)=Xe : Product  Inputs=3  SaturateOnIntegerOverflow=on  InputSameDT=on
  (Rh+h)cos(phi)*sin(lamb)=Ye : Product  Inputs=3  SaturateOnIntegerOverflow=on  InputSameDT=on
  Deg2R : Gain  Gain=pi/180  SaturateOnIntegerOverflow=on
  "Deg2R " : Gain  Gain=pi/180  SaturateOnIntegerOverflow=on
  Product1 : Product  SaturateOnIntegerOverflow=on  InputSameDT=on
  Re=equatorial radius : Constant  Value=Re
  Rh : Product  Inputs=*/  SaturateOnIntegerOverflow=on  InputSameDT=on
  Rh(1-e^2) : Product  SaturateOnIntegerOverflow=on  InputSameDT=on
  Sum1 : Sum  Inputs=+-|  SaturateOnIntegerOverflow=on  InputSameDT=on
  Sum2 : Sum  SaturateOnIntegerOverflow=on  InputSameDT=on
      settings: AttributesFormatString=Rh+h
  Sum3 : Sum  Inputs=|+-  SaturateOnIntegerOverflow=on  InputSameDT=on
  Sum4 : Sum  SaturateOnIntegerOverflow=on  InputSameDT=on
      settings: AttributesFormatString=(1-e^2)Rh+h
  Ze : Product  SaturateOnIntegerOverflow=on  InputSameDT=on
  const : Constant
  const1 : Constant
  cos(lamb) : Trigonometry  Operator=cos
  cos(phi) : Trigonometry  Operator=cos
  eccentricity^2 : Subsystem
  f : Fcn  Expr=sqrt(u(1))
  sin(lamb) : Trigonometry
  sin(phi) : Trigonometry
  sin(phi)^2 : Product  SaturateOnIntegerOverflow=on  InputSameDT=on
  "Xe, m " : Outport
  "Ye, m " : Outport  Port=2
  "Ze, m " : Outport  Port=3
  wires:
  "lat, deg"/1 -> Deg2R/1
  sin(phi)/1 -> sin(phi)^2/1, sin(phi)^2/2, Ze/1
  f/1 -> Rh/2
  Re=equatorial radius/1 -> Rh/1
  Rh/1 -> Sum2/2, Rh(1-e^2)/2
  Product1/1 -> Sum1/2
  Sum1/1 -> f/1
  const/1 -> Sum1/1
  "height, m"/1 -> Sum4/2, Sum2/1
  eccentricity^2/1(e^2) -> Product1/1, Sum3/2
  sin(phi)^2/1 -> Product1/2
  const1/1 -> Sum3/1
  Sum3/1 -> Rh(1-e^2)/1  "1-e^2"
  Rh(1-e^2)/1 -> Sum4/1
  Sum4/1 -> Ze/2
  lon,deg/1 -> "Deg2R "/1
  cos(phi)/1 -> (Rh+h)cos(phi)*cos(lamb)=Xe/2, (Rh+h)cos(phi)*sin(lamb)=Ye/2
  cos(lamb)/1 -> (Rh+h)cos(phi)*cos(lamb)=Xe/3
  sin(lamb)/1 -> (Rh+h)cos(phi)*sin(lamb)=Ye/3
  Ze/1 -> "Ze, m "/1
  Deg2R/1 -> cos(phi)/1, sin(phi)/1
  "Deg2R "/1 -> cos(lamb)/1, sin(lamb)/1
  Sum2/1 -> (Rh+h)cos(phi)*sin(lamb)=Ye/1, (Rh+h)cos(phi)*cos(lamb)=Xe/1
  (Rh+h)cos(phi)*cos(lamb)=Xe/1 -> "Xe, m "/1
  (Rh+h)cos(phi)*sin(lamb)=Ye/1 -> "Ye, m "/1

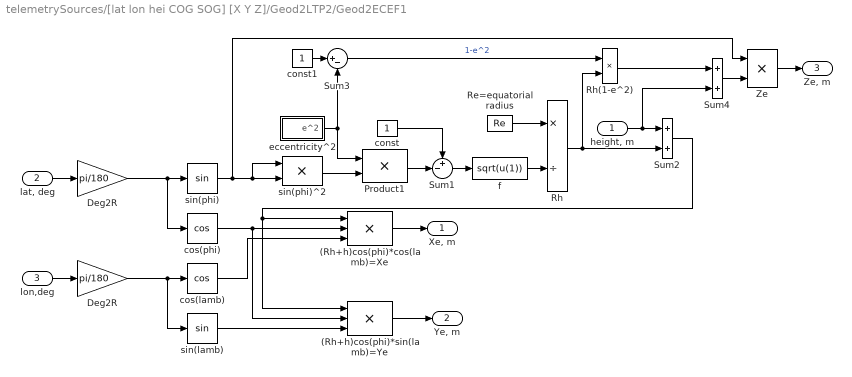
== system telemetrySources/[lat lon hei COG SOG] [X Y Z]/Geod2LTP2/Geod2ECEF1 ==
  "height, m" : Inport
  "lat, deg" : Inport  Port=2
  lon,deg : Inport  Port=3
  (Rh+h)cos(phi)*cos(lamb)=Xe : Product  Inputs=3  SaturateOnIntegerOverflow=on  InputSameDT=on
  (Rh+h)cos(phi)*sin(lamb)=Ye : Product  Inputs=3  SaturateOnIntegerOverflow=on  InputSameDT=on
  Deg2R : Gain  Gain=pi/180  SaturateOnIntegerOverflow=on
  "Deg2R " : Gain  Gain=pi/180  SaturateOnIntegerOverflow=on
  Product1 : Product  SaturateOnIntegerOverflow=on  InputSameDT=on
  Re=equatorial radius : Constant  Value=Re
  Rh : Product  Inputs=*/  SaturateOnIntegerOverflow=on  InputSameDT=on
  Rh(1-e^2) : Product  SaturateOnIntegerOverflow=on  InputSameDT=on
  Sum1 : Sum  Inputs=+-|  SaturateOnIntegerOverflow=on  InputSameDT=on
  Sum2 : Sum  SaturateOnIntegerOverflow=on  InputSameDT=on
      settings: AttributesFormatString=Rh+h
  Sum3 : Sum  Inputs=|+-  SaturateOnIntegerOverflow=on  InputSameDT=on
  Sum4 : Sum  SaturateOnIntegerOverflow=on  InputSameDT=on
      settings: AttributesFormatString=(1-e^2)Rh+h
  Ze : Product  SaturateOnIntegerOverflow=on  InputSameDT=on
  const : Constant
  const1 : Constant
  cos(lamb) : Trigonometry  Operator=cos
  cos(phi) : Trigonometry  Operator=cos
  eccentricity^2 : Subsystem
  f : Fcn  Expr=sqrt(u(1))
  sin(lamb) : Trigonometry
  sin(phi) : Trigonometry
  sin(phi)^2 : Product  SaturateOnIntegerOverflow=on  InputSameDT=on
  "Xe, m " : Outport
  "Ye, m " : Outport  Port=2
  "Ze, m " : Outport  Port=3
  wires:
  (Rh+h)cos(phi)*sin(lamb)=Ye/1 -> "Ye, m "/1
  (Rh+h)cos(phi)*cos(lamb)=Xe/1 -> "Xe, m "/1
  Sum2/1 -> (Rh+h)cos(phi)*cos(lamb)=Xe/1, (Rh+h)cos(phi)*sin(lamb)=Ye/1
  "Deg2R "/1 -> sin(lamb)/1, cos(lamb)/1
  Deg2R/1 -> sin(phi)/1, cos(phi)/1
  Ze/1 -> "Ze, m "/1
  sin(lamb)/1 -> (Rh+h)cos(phi)*sin(lamb)=Ye/3
  cos(lamb)/1 -> (Rh+h)cos(phi)*cos(lamb)=Xe/3
  cos(phi)/1 -> (Rh+h)cos(phi)*sin(lamb)=Ye/2, (Rh+h)cos(phi)*cos(lamb)=Xe/2
  lon,deg/1 -> "Deg2R "/1
  Sum4/1 -> Ze/2
  Rh(1-e^2)/1 -> Sum4/1
  Sum3/1 -> Rh(1-e^2)/1  "1-e^2"
  const1/1 -> Sum3/1
  sin(phi)^2/1 -> Product1/2
  eccentricity^2/1(e^2) -> Sum3/2, Product1/1
  "height, m"/1 -> Sum2/1, Sum4/2
  const/1 -> Sum1/1
  Sum1/1 -> f/1
  Product1/1 -> Sum1/2
  Rh/1 -> Rh(1-e^2)/2, Sum2/2
  Re=equatorial radius/1 -> Rh/1
  f/1 -> Rh/2
  sin(phi)/1 -> Ze/1, sin(phi)^2/2, sin(phi)^2/1
  "lat, deg"/1 -> Deg2R/1

== system telemetrySources/Static/Baro Altimeter/Initial Baro Bias/Low Pass8 ==
  In1 : Inport
  Discrete Zero-Pole : DiscreteZeroPole  Zeros=zerosd  Poles=polesd  Gain=gaind  SampleTime=SampleTime
  Out1 : Outport
  wires:
  In1/1 -> Discrete Zero-Pole/1
  Discrete Zero-Pole/1 -> Out1/1

== system telemetrySources/[lat lon hei COG SOG] [X Y Z]/Geod2LTP2/ECEF2LTP (UEN)/From Body to Universal1 ==
  long : Inport
  lat : Inport  Port=2
  Mux : Mux  Inputs=2
  Reshape 9x1->3x1 : S-Function  FunctionName=sreshape  Parameters=OutputDimensionality, OutputDimensions  mask(Reshape){OutputDimensionality=Customize, OutputDimensions=[3,3]}
      mask prompts: OutputDimensionality "Output dimensionality:"; OutputDimensions "Output dimensions:"
      mask help:
      | Change the dimensions of a vector or matrix input signal. Output
      |  - a one-dimensional array (vector),
      |  - a column vector (Mx1 matrix),
      |  - a row vector (1xN matrix), or
      |  - a matrix or vector with specified dimensions, e.g., [M, N] or [W].
      mask init:
      | s = reshapemask(gcb,'init');
      mask StyleString: popup(1-D array|Column vector|Row vector|Customize),edit
      mask CallbackString: reshapemask(gcb,'cbDimensionality')|
      mask Display: disp('Reshape')
  Rotation Matrix from Long//Lat : Subsystem
      mask Type: Vector Transformation
      mask Description: Vector Transformation
      mask Display: disp('axis')
  DCM : Outport
  wires:
  lat/1 -> Mux/2
  long/1 -> Mux/1
  Mux/1 -> Rotation Matrix from Long//Lat/1(long lat)
  Rotation Matrix from Long//Lat/1(DCM) -> Reshape 9x1->3x1/1
  Reshape 9x1->3x1/1 -> DCM/1

== system telemetrySources/[lat lon hei COG SOG] [X Y Z]/Geod2LTP2/Geod2ECEF/eccentricity^2 ==
  " " : Product  SaturateOnIntegerOverflow=on  InputSameDT=on
  Re=equatorial radius1 : Constant  Value=Re
  Rp=polar radius : Constant  Value=Rp
  Sum5 : Sum  Inputs=|+-  SaturateOnIntegerOverflow=on  InputSameDT=on
  const2 : Constant
  e^1 : Product  Inputs=*/  SaturateOnIntegerOverflow=on  InputSameDT=on
  e^2 : Outport
  wires:
  Re=equatorial radius1/1 -> e^1/2
  Rp=polar radius/1 -> e^1/1
  const2/1 -> Sum5/1
  e^1/1 -> " "/2, " "/1
  " "/1 -> Sum5/2
  Sum5/1 -> e^2/1

== system telemetrySources/[lat lon hei COG SOG] [X Y Z]/Geod2LTP2/Geod2ECEF1/eccentricity^2 ==
  " " : Product  SaturateOnIntegerOverflow=on  InputSameDT=on
  Re=equatorial radius1 : Constant  Value=Re
  Rp=polar radius : Constant  Value=Rp
  Sum5 : Sum  Inputs=|+-  SaturateOnIntegerOverflow=on  InputSameDT=on
  const2 : Constant
  e^1 : Product  Inputs=*/  SaturateOnIntegerOverflow=on  InputSameDT=on
  e^2 : Outport
  wires:
  Sum5/1 -> e^2/1
  " "/1 -> Sum5/2
  e^1/1 -> " "/1, " "/2
  const2/1 -> Sum5/1
  Rp=polar radius/1 -> e^1/1
  Re=equatorial radius1/1 -> e^1/2

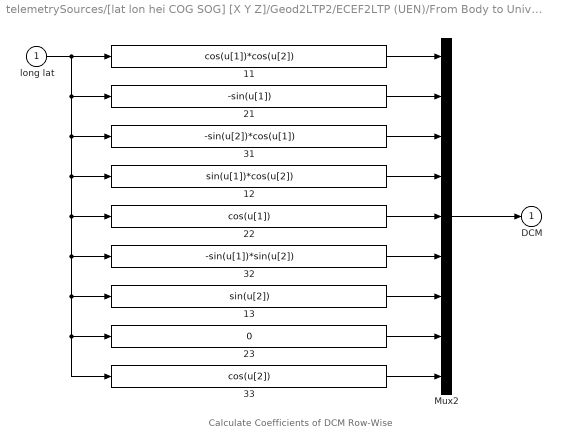
== system telemetrySources/[lat lon hei COG SOG] [X Y Z]/Geod2LTP2/ECEF2LTP (UEN)/From Body to Universal1/Rotation Matrix from Long//Lat ==
  note: Calculate Coefficients of DCM Row-Wise
  long lat : Inport
  11 : Fcn  Expr=cos(u[1])*cos(u[2])
  12 : Fcn  Expr=sin(u[1])*cos(u[2])
  13 : Fcn  Expr=sin(u[2])
  21 : Fcn  Expr=-sin(u[1])
  22 : Fcn  Expr=cos(u[1])
  23 : Fcn  Expr=0
  31 : Fcn  Expr=-sin(u[2])*cos(u[1])
  32 : Fcn  Expr=-sin(u[1])*sin(u[2])
  33 : Fcn  Expr=cos(u[2])
  Mux2 : Mux  Inputs=9
  DCM : Outport  InitialOutput=0
  wires:
  33/1 -> Mux2/9
  23/1 -> Mux2/8
  13/1 -> Mux2/7
  32/1 -> Mux2/6
  22/1 -> Mux2/5
  12/1 -> Mux2/4
  31/1 -> Mux2/3
  21/1 -> Mux2/2
  11/1 -> Mux2/1
  Mux2/1 -> DCM/1
  long lat/1 -> 11/1, 33/1, 23/1, 13/1, 32/1, 22/1, 12/1, 31/1, 21/1

== matlab function Magnetic Field/3D Filter/myMux Fun1 ==
  data: u1 input inherited; y output inherited; u2 input inherited; u3 input inherited
function y = myMux(u1, u2, u3)
% This block supports an embeddable subset of the MATLAB language.
% See the help menu for details. 

y = [u1(1); u2(1); u3(1)];

== matlab function Static/Baro Altimeter/Enables/Disables the Computation of initial Baro Bias ==
  data: tOut output inherited
function tOut = getTIni

persistent aveCount;
persistent tIni;

if isempty(aveCount)
    aveCount =1;
    tIni = 1;
end;

if aveCount < 2500
    aveCount = aveCount + 1;
end

if aveCount == 2500
    tIni =0;
    aveCount = aveCount + 1;
end

tOut = tIni;

%if aveCount > 500
%    tIni = 0;
%end

% if isempty(aveCount)
%     aveCount =1;
%     initBias = [0.0 0.0 0.0]';
% end;
%     
% if (aveCount<10)
%     initBias = initBias+ Raw;
%     bias = initBias/aveCount;
%     aveCount = aveCount +1;
% end;
% 
% if (aveCount == 10)
%     initBias = initBias/(aveCount-1);
%     aveCount = 100;
% end;
% 
% if (aveCount == 100)
%     bias = initBias;
% end;
